simulink model "Synch_gen_model_full_order"  (R2013a)
settings: Solver=ode23tb  StartTime=0.0  StopTime=10  FixedStep=0.01  MaxStep=0.0005  RelTol=1e-5  AbsTol=1e-4
values from neighbouring files (symbols this model uses):
  D = 0    [Gen_Init_SynFull_Order.m]
  deltag0 = angle(Uq0bar)    [Gen_Init_SynFull_Order.m]
  H = 2.86    [Gen_Init_SynFull_Order.m]
  Ra = 0.01    [Gen_Init_SynFull_Order.m]
  RL = uqg0/iq0    [Gen_Init_SynFull_Order.m]
  sid0 = xd*id0+Ufd0    [Gen_Init_SynFull_Order.m]
  sif0 = sid0 + (xdd/(xd-xdd))*Ufd0    [Gen_Init_SynFull_Order.m]
  sig0 = siq0    [Gen_Init_SynFull_Order.m]
  SigmaInv = 1/0.05    (= 20)    [Gen_Init_SynFull_Order.m]
  sih0 = sid0    [Gen_Init_SynFull_Order.m]
  sik0 = siq0    [Gen_Init_SynFull_Order.m]
  siq0 = xq*iq0    [Gen_Init_SynFull_Order.m]
  Tdd = 0.4    [Gen_Init_SynFull_Order.m]
  Tddd = 0.0259    [Gen_Init_SynFull_Order.m]
  Tm = Te0    [Gen_Init_SynFull_Order.m]
  Tqd = 0.1073    [Gen_Init_SynFull_Order.m]
  Tqdd = 0.0463    [Gen_Init_SynFull_Order.m]
  Tswitch = input('Enter the time at which Genarator is synchronized: ')    [Gen_Init_SynFull_Order.m]
  Ufd0 = Uq0-(xd-xq)*id0    [Gen_Init_SynFull_Order.m]
  w0 = 50*2*pi    (= 314.159265359)    [Gen_Init_SynFull_Order.m]
  W0init = 1    [Gen_Init_SynFull_Order.m]
  wB = 50*2*pi    (= 314.159265359)    [Gen_Init_SynFull_Order.m]
  xd = 1.79    [Gen_Init_SynFull_Order.m]
  xdd = 0.169    [Gen_Init_SynFull_Order.m]
  xddd = 0.135    [Gen_Init_SynFull_Order.m]
  xfl = (xd*xdd)/(xd-xdd)    (= 0.186619370759)    [Gen_Init_SynFull_Order.m]
  xq = 1.71    [Gen_Init_SynFull_Order.m]
  xqd = 0.228    [Gen_Init_SynFull_Order.m]
  xqdd = 0.2    [Gen_Init_SynFull_Order.m]
  Ymat = inv(Zmat)    [Gen_Init_SynFull_Order.m]
settings Model: Creator=Korai  LastModifiedBy=Korai
settings RTWCC: TargetLang=C++

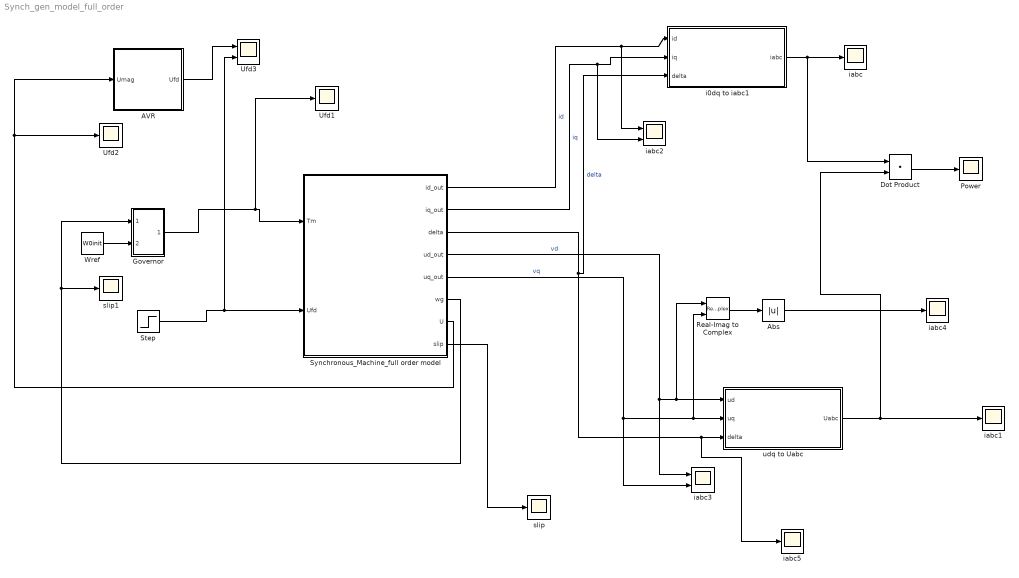
== system Synch_gen_model_full_order ==
  AVR : Subsystem
  Abs : Abs
  Dot Product : DotProduct  InputSameDT=on  OutDataTypeStr=Inherit: Inherit via internal rule
  Governor : Subsystem
  Power : Scope
      settings: YMin=0.0095  YMax=0.0105  SaveName=ScopeData5
  Real-Imag to Complex : RealImagToComplex
  Step : Step  Time=0  After=Ufd0  SampleTime=0
  Synchronous_Machine_full order model : Subsystem
  Ufd1 : Scope
      settings: YMin=-0.55  YMax=0.55  SaveName=ScopeData11
  Ufd2 : Scope
      settings: SaveName=ScopeData13
  Ufd3 : Scope  NumInputPorts=2
      settings: YMin=-3e-05~1.03987  YMax=2.25e-05~1.14933  SaveName=ScopeData16
  Wref : Constant  Value=W0init
  i0dq to iabc1 : Subsystem
  iabc{,1,4..5} (4 alike) : Scope
      iabc settings: YMin=-7  YMax=7
      iabc1 settings: YMin=-0.9  YMax=0.9  SaveName=ScopeData2
      iabc4 settings: YMin=0.95  YMax=1.05  SaveName=ScopeData23
      iabc5 settings: YMin=-0.9  YMax=0.9  SaveName=ScopeData25
  iabc2 : Scope  NumInputPorts=2
      settings: ShowLegends=on  YMin=-0.0004865~0.02665  YMax=-0.000475~0.0272  SaveName=ScopeData9
  iabc3 : Scope  NumInputPorts=2
      settings: ShowLegends=on  YMin=-0.0184~0.99983  YMax=-0.0166~0.999862  SaveName=ScopeData10
  slip : Scope
      settings: SaveName=ScopeData12
  slip1 : Scope
      settings: SaveName=ScopeData24
  udq to Uabc : Subsystem
  wires:
  i0dq to iabc1/1(iabc) -> iabc/1, Dot Product/1
  udq to Uabc/1(Uabc) -> Dot Product/2, iabc1/1
  Dot Product/1 -> Power/1
  Synchronous_Machine_full order model/3(delta) -> i0dq to iabc1/3(delta), iabc5/1, udq to Uabc/3(delta)  "delta"
  Synchronous_Machine_full order model/1(id_out) -> i0dq to iabc1/1(id), iabc2/1  "id"
  Synchronous_Machine_full order model/2(iq_out) -> i0dq to iabc1/2(iq), iabc2/2  "iq"
  Synchronous_Machine_full order model/4("ud_out ") -> Real-Imag to Complex/1, udq to Uabc/1(ud), iabc3/1  "vd"
  Synchronous_Machine_full order model/5(uq_out) -> Real-Imag to Complex/2, udq to Uabc/2(uq), iabc3/2  "vq"
  Synchronous_Machine_full order model/6(wg) -> slip1/1, Governor/1(wpu)
  Wref/1 -> Governor/2(w_ref)
  Synchronous_Machine_full order model/7(U) -> AVR/1(Umag), Ufd2/1
  Synchronous_Machine_full order model/8(slip) -> slip/1
  Governor/1(Tm) -> Ufd1/1, Synchronous_Machine_full order model/1(Tm)
  Real-Imag to Complex/1 -> Abs/1
  Abs/1 -> iabc4/1
  AVR/1(Ufd) -> Ufd3/1
  Step/1 -> Ufd3/2, Synchronous_Machine_full order model/2(Ufd)

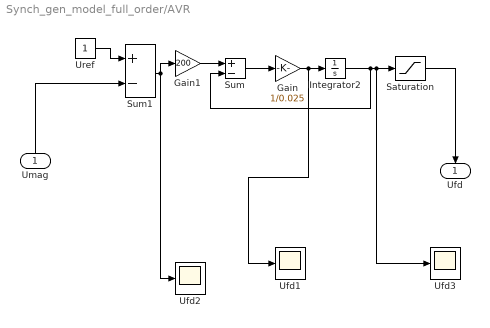
== system Synch_gen_model_full_order/AVR ==
  Umag : Inport
  Gain : Gain  Gain=1/0.025  SaturateOnIntegerOverflow=on  OutDataTypeStr=Inherit: Same as input  ParamDataTypeStr=Inherit: Same as input
  Gain1 : Gain  Gain=200  SaturateOnIntegerOverflow=on  OutDataTypeStr=Inherit: Same as input  ParamDataTypeStr=Inherit: Same as input
  Integrator2 : Integrator  InitialCondition=Ufd0
  Saturation : Saturate  UpperLimit=6  LowerLimit=-6
  Sum : Sum  Inputs=+-  SaturateOnIntegerOverflow=on  InputSameDT=on  OutDataTypeStr=Inherit: Same as first input
  Sum1 : Sum  Inputs=+-  SaturateOnIntegerOverflow=on  InputSameDT=on  OutDataTypeStr=Inherit: Same as first input
  Ufd1 : Scope
      settings: YMin=-550  YMax=550  SaveName=ScopeData19
  Ufd2 : Scope
      settings: YMin=-0.08  YMax=0.07  SaveName=ScopeData20
  Ufd3 : Scope
      settings: YMin=-2.75  YMax=1  SaveName=ScopeData18
  Uref : Constant
  Ufd : Outport
  wires:
  Gain/1 -> Ufd1/1, Integrator2/1
  Saturation/1 -> Ufd/1
  Sum/1 -> Gain/1
  Uref/1 -> Sum1/1
  Gain1/1 -> Sum/1
  Integrator2/1 -> Sum/2, Ufd3/1, Saturation/1
  Sum1/1 -> Gain1/1, Ufd2/1
  Umag/1 -> Sum1/2

== system Synch_gen_model_full_order/Governor ==
  wpu : Inport
  w_ref : Inport  Port=2
  Gain : Gain  Gain=1/0.01  SaturateOnIntegerOverflow=on  OutDataTypeStr=Inherit: Same as input  ParamDataTypeStr=Inherit: Same as input
  Gain15 : Gain  Gain=SigmaInv  SaturateOnIntegerOverflow=on  OutDataTypeStr=Inherit: Same as input  ParamDataTypeStr=Inherit: Same as input
  Integrator : Integrator  InitialCondition=Tm
  Sum : Sum  Inputs=+-  SaturateOnIntegerOverflow=on  InputSameDT=on  OutDataTypeStr=Inherit: Same as first input
  Sum1 : Sum  SaturateOnIntegerOverflow=on  InputSameDT=on  OutDataTypeStr=Inherit: Same as first input
  Sum8 : Sum  Inputs=+-  SaturateOnIntegerOverflow=on  InputSameDT=on  OutDataTypeStr=Inherit: Same as first input
  Tm0 : Constant  Value=Tm
  Tm : Outport
  wires:
  w_ref/1 -> Sum8/1
  Sum8/1 -> Gain15/1
  wpu/1 -> Sum8/2
  Sum/1 -> Gain/1
  Gain/1 -> Integrator/1
  Integrator/1 -> Sum/2, Tm/1
  Gain15/1 -> Sum1/2
  Sum1/1 -> Sum/1
  Tm0/1 -> Sum1/1

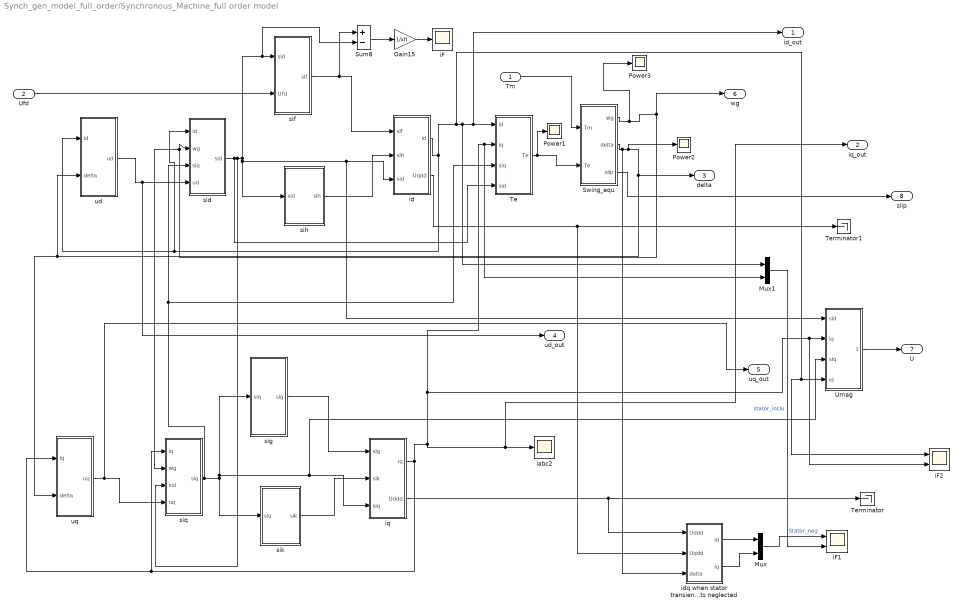
== system Synch_gen_model_full_order/Synchronous_Machine_full order model ==
  Tm : Inport
  Ufd : Inport  Port=2
  Gain15 : Gain  Gain=1/xfl  SaturateOnIntegerOverflow=on  OutDataTypeStr=Inherit: Same as input  ParamDataTypeStr=Inherit: Same as input
  Mux : Mux  Inputs=2
  Mux1 : Mux  Inputs=2
  Power1 : Scope
      settings: YMin=0.010195  YMax=0.01023  SaveName=ScopeData6
  Power2 : Scope
      settings: YMin=0.82  YMax=0.885  SaveName=ScopeData7
  Power3 : Scope
      settings: YMin=0.95  YMax=1.05  SaveName=ScopeData8
  Sum8 : Sum  Inputs=+-  SaturateOnIntegerOverflow=on  InputSameDT=on  OutDataTypeStr=Inherit: Same as first input
  "Swing_equ " : Subsystem
  Te : Subsystem
  Terminator : Terminator
  Terminator1 : Terminator
  Umag : Subsystem
  iF : Scope
      settings: SaveName=ScopeData4
  iF1 : Scope  NumInputPorts=2
      settings: ShowLegends=on  YMin=-17.5~-25  YMax=7.5~12.5  SaveName=ScopeData14
  iF2 : Scope  NumInputPorts=2
      settings: YMin=-0.191~0.190025  YMax=-0.189~0.1905  SaveName=ScopeData15
  iabc2 : Scope
      settings: YMin=0.0054  YMax=0.00645  SaveName=ScopeData3
  id : Subsystem
  idq when stator transients neglected : Subsystem
  iq : Subsystem
  sid : Subsystem
  sif : Subsystem
  sig : Subsystem
  sih : Subsystem
  sik : Subsystem
  siq : Subsystem
  ud : Subsystem
  uq : Subsystem
  id_out : Outport
  iq_out : Outport  Port=2
  delta : Outport  Port=3
  "ud_out " : Outport  Port=4
  uq_out : Outport  Port=5
  wg : Outport  Port=6
  U : Outport  Port=7
  slip : Outport  Port=8
  wires:
  iq/2(Uddd) -> idq when stator transients neglected/1(Uddd), Terminator/1
  id/1(id) -> Umag/4(id), iF2/1, Mux1/1, id_out/1, Te/1(id), sid/1(id), ud/1(id)
  sif/1(sif) -> Sum8/1, id/1(sif)
  sih/1(sih) -> id/2(sih)
  sid/1(sid) -> Te/4(sid), siq/3(sid), Sum8/2, sif/1(sid), sih/1(sid), Umag/1(sid), id/3(sid)
  iq/1(iq) -> uq/1(iq), siq/1(iq), Mux1/2, Te/2(iq), iF2/2, Umag/2(iq), iq_out/1, iabc2/1
  Gain15/1 -> iF/1
  Tm/1 -> "Swing_equ "/1(Tm)
  Sum8/1 -> Gain15/1
  id/2(Uqdd) -> Terminator1/1, idq when stator transients neglected/2(Uqdd)
  sik/1(sik) -> iq/2(sik)
  Te/1(Te) -> "Swing_equ "/2(Te), Power1/1
  "Swing_equ "/1(wg) -> Power3/1, siq/2(wg), sid/2(wg), wg/1
  "Swing_equ "/2(delta) -> idq when stator transients neglected/3(delta), Power2/1, delta/1, uq/2(delta), ud/2(delta)
  sig/1(sig) -> iq/1(sig)
  siq/1(siq) -> Te/3(siq), sid/3(siq), Umag/3(siq), iq/3(siq), sig/1(siq), sik/1(siq)
  Ufd/1 -> sif/2(Ufd)
  Umag/1(Umag) -> U/1
  "Swing_equ "/3(slip) -> slip/1
  ud/1(ud) -> "ud_out "/1, sid/4(ud)
  uq/1(uq) -> uq_out/1, siq/4(uq)
  idq when stator transients neglected/1(id) -> Mux/1
  idq when stator transients neglected/2(iq) -> Mux/2
  Mux/1 -> iF1/1  "Stator_neg"
  Mux1/1 -> iF1/2  "stator_inclu"

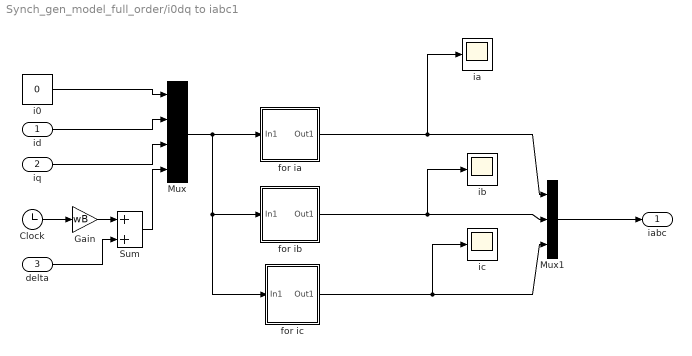
== system Synch_gen_model_full_order/i0dq to iabc1 ==
  id : Inport
  iq : Inport  Port=2
  delta : Inport  Port=3
  Clock : Clock
  Gain : Gain  Gain=wB  SaturateOnIntegerOverflow=on  OutDataTypeStr=Inherit: Same as input  ParamDataTypeStr=Inherit: Same as input
  Mux : Mux
  Mux1 : Mux  Inputs=3
  Sum : Sum  Inputs=|++  SaturateOnIntegerOverflow=on  InputSameDT=on  OutDataTypeStr=Inherit: Same as first input
  for ia : Subsystem
  for ib : Subsystem
  for ic : Subsystem
  i0 : Constant  Value=0
  ia : Scope
  ib : Scope
  ic : Scope
  iabc : Outport
  wires:
  i0/1 -> Mux/1
  Sum/1 -> Mux/4
  Clock/1 -> Gain/1
  Gain/1 -> Sum/1
  delta/1 -> Sum/2
  Mux/1 -> for ic/1(In1), for ib/1(In1), for ia/1(In1)
  Mux1/1 -> iabc/1
  iq/1 -> Mux/3
  id/1 -> Mux/2
  for ic/1(Out1) -> ic/1, Mux1/3
  for ib/1(Out1) -> ib/1, Mux1/2
  for ia/1(Out1) -> ia/1, Mux1/1

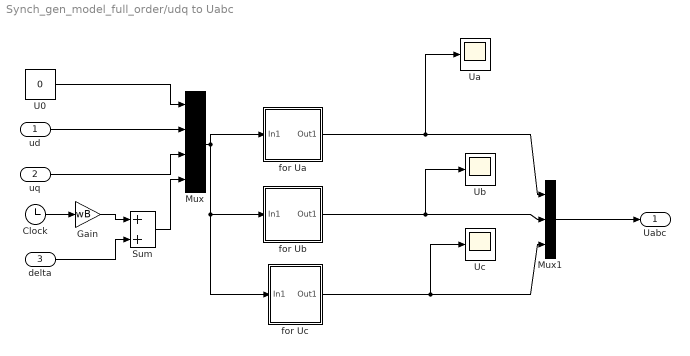
== system Synch_gen_model_full_order/udq to Uabc ==
  ud : Inport
  uq : Inport  Port=2
  delta : Inport  Port=3
  Clock : Clock
  Gain : Gain  Gain=wB  SaturateOnIntegerOverflow=on  OutDataTypeStr=Inherit: Same as input  ParamDataTypeStr=Inherit: Same as input
  Mux : Mux
  Mux1 : Mux  Inputs=3
  Sum : Sum  Inputs=|++  SaturateOnIntegerOverflow=on  InputSameDT=on  OutDataTypeStr=Inherit: Same as first input
  U0 : Constant  Value=0
  Ua : Scope
  Ub : Scope
  Uc : Scope
  for Ua : Subsystem
  for Ub : Subsystem
  for Uc : Subsystem
  Uabc : Outport
  wires:
  for Ua/1(Out1) -> Mux1/1, Ua/1
  for Ub/1(Out1) -> Mux1/2, Ub/1
  for Uc/1(Out1) -> Mux1/3, Uc/1
  U0/1 -> Mux/1
  ud/1 -> Mux/2
  uq/1 -> Mux/3
  Mux1/1 -> Uabc/1
  delta/1 -> Sum/2
  Clock/1 -> Gain/1
  Gain/1 -> Sum/1
  Sum/1 -> Mux/4
  Mux/1 -> for Ua/1(In1), for Ub/1(In1), for Uc/1(In1)

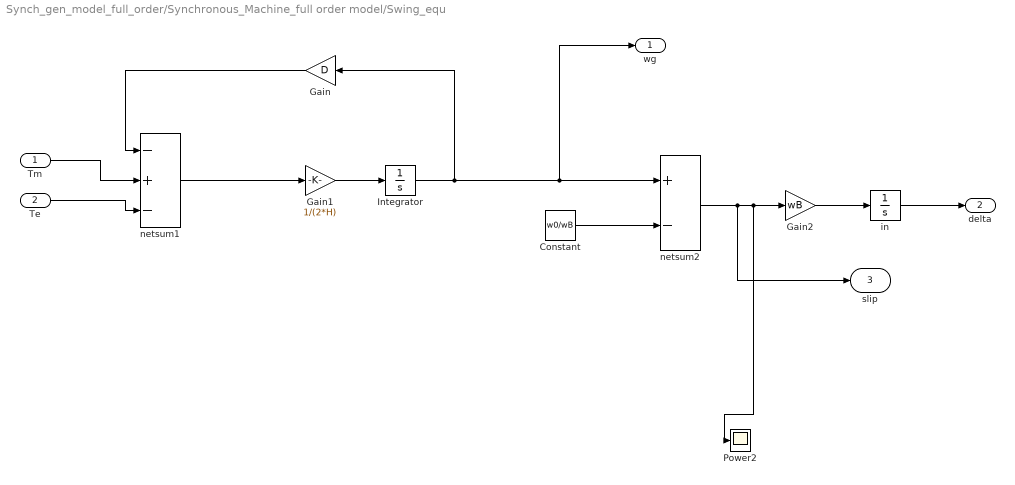
== system Synch_gen_model_full_order/Synchronous_Machine_full order model/Swing_equ  ==
  Tm : Inport
  Te : Inport  Port=2
  Constant : Constant  Value=w0/wB
  Gain : Gain  Gain=D
  Gain1 : Gain  Gain=1/(2*H)
  Gain2 : Gain  Gain=wB  SaturateOnIntegerOverflow=on  OutDataTypeStr=Inherit: Same as input  ParamDataTypeStr=Inherit: Same as input
  Integrator : Integrator  InitialCondition=W0init
  Power2 : Scope
      settings: YMin=0.82  YMax=0.885  SaveName=ScopeData26
  in : Integrator  InitialCondition=deltag0
  netsum1 : Sum  Inputs=-+-  SaturateOnIntegerOverflow=on  InputSameDT=on  OutDataTypeStr=Inherit: Same as first input
  netsum2 : Sum  Inputs=+-  SaturateOnIntegerOverflow=on  InputSameDT=on  OutDataTypeStr=Inherit: Same as first input
  wg : Outport
  delta : Outport  Port=2
  slip : Outport  Port=3
  wires:
  Te/1 -> netsum1/3
  Tm/1 -> netsum1/2
  Gain/1 -> netsum1/1
  netsum1/1 -> Gain1/1
  Gain1/1 -> Integrator/1
  Integrator/1 -> netsum2/1, wg/1, Gain/1
  Constant/1 -> netsum2/2
  Gain2/1 -> in/1
  in/1 -> delta/1
  netsum2/1 -> slip/1, Power2/1, Gain2/1

== system Synch_gen_model_full_order/Synchronous_Machine_full order model/Te ==
  id : Inport
  iq : Inport  Port=2
  siq : Inport  Port=3
  sid : Inport  Port=4
  Product : Product
  Product1 : Product
  netsum : Sum  Inputs=+-  SaturateOnIntegerOverflow=on  InputSameDT=on  OutDataTypeStr=Inherit: Same as first input
  Te : Outport
  wires:
  netsum/1 -> Te/1
  sid/1 -> Product/1
  iq/1 -> Product/2
  Product/1 -> netsum/1
  id/1 -> Product1/1
  siq/1 -> Product1/2
  Product1/1 -> netsum/2

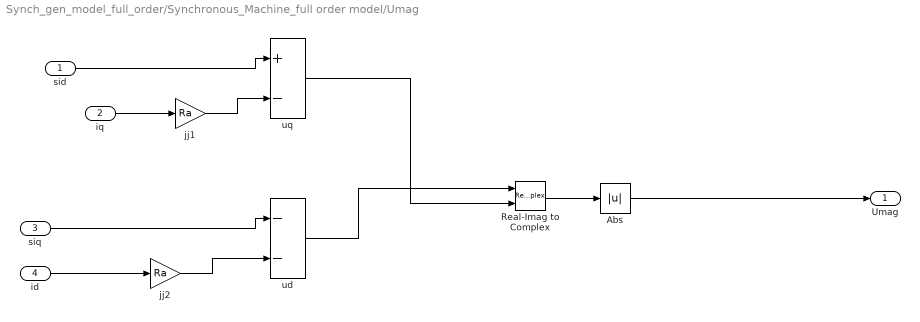
== system Synch_gen_model_full_order/Synchronous_Machine_full order model/Umag ==
  sid : Inport
  iq : Inport  Port=2
  siq : Inport  Port=3
  id : Inport  Port=4
  Abs : Abs
  Real-Imag to Complex : RealImagToComplex
  jj1 : Gain  Gain=Ra
  jj2 : Gain  Gain=Ra
  ud : Sum  Inputs=--  SaturateOnIntegerOverflow=on  InputSameDT=on  OutDataTypeStr=Inherit: Same as first input
  uq : Sum  Inputs=+-  SaturateOnIntegerOverflow=on  InputSameDT=on  OutDataTypeStr=Inherit: Same as first input
  Umag : Outport
  wires:
  sid/1 -> uq/1
  Abs/1 -> Umag/1
  iq/1 -> jj1/1
  jj1/1 -> uq/2
  siq/1 -> ud/1
  id/1 -> jj2/1
  jj2/1 -> ud/2
  uq/1 -> Real-Imag to Complex/2
  ud/1 -> Real-Imag to Complex/1
  Real-Imag to Complex/1 -> Abs/1

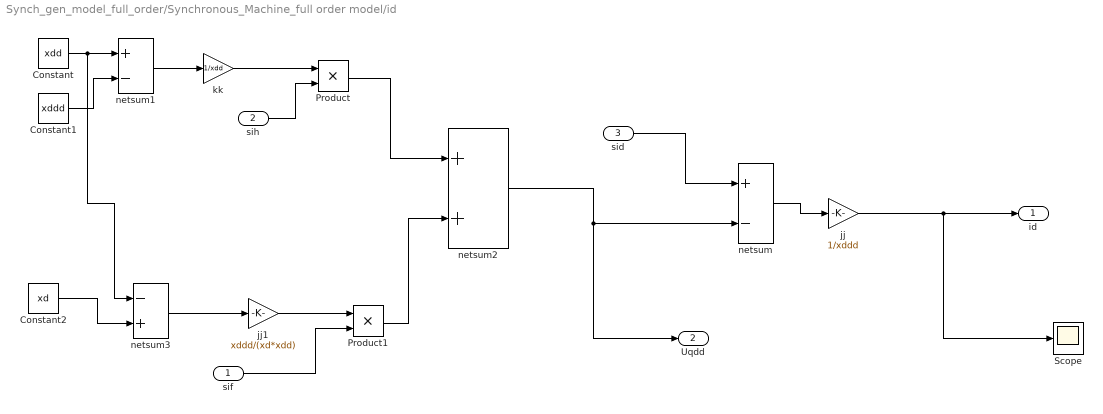
== system Synch_gen_model_full_order/Synchronous_Machine_full order model/id ==
  sif : Inport
  sih : Inport  Port=2
  sid : Inport  Port=3
  Constant : Constant  Value=xdd
  Constant1 : Constant  Value=xddd
  Constant2 : Constant  Value=xd
  Product : Product
  Product1 : Product
  Scope : Scope
      settings: SaveName=ScopeData29
  jj : Gain  Gain=1/xddd
  jj1 : Gain  Gain=xddd/(xd*xdd)
  kk : Gain  Gain=1/xdd
  netsum : Sum  Inputs=+-  SaturateOnIntegerOverflow=on  InputSameDT=on  OutDataTypeStr=Inherit: Same as first input
  netsum1 : Sum  Inputs=+-  SaturateOnIntegerOverflow=on  InputSameDT=on  OutDataTypeStr=Inherit: Same as first input
  netsum2 : Sum  SaturateOnIntegerOverflow=on  InputSameDT=on  OutDataTypeStr=Inherit: Same as first input
  netsum3 : Sum  Inputs=-+  SaturateOnIntegerOverflow=on  InputSameDT=on  OutDataTypeStr=Inherit: Same as first input
  id : Outport
  Uqdd : Outport  Port=2
  wires:
  Constant/1 -> netsum3/1, netsum1/1
  Constant1/1 -> netsum1/2
  netsum1/1 -> kk/1
  kk/1 -> Product/1
  sih/1 -> Product/2
  Product/1 -> netsum2/1
  Constant2/1 -> netsum3/2
  netsum3/1 -> jj1/1
  jj1/1 -> Product1/1
  sif/1 -> Product1/2
  Product1/1 -> netsum2/2
  netsum2/1 -> netsum/2, Uqdd/1
  sid/1 -> netsum/1
  netsum/1 -> jj/1
  jj/1 -> Scope/1, id/1

== system Synch_gen_model_full_order/Synchronous_Machine_full order model/idq when stator transients neglected ==
  Uddd : Inport
  Uqdd : Inport  Port=2
  delta : Inport  Port=3
  Demux : Demux  Outputs=2
  Mux1 : Mux  Inputs=2
  Synchronize : Subsystem
  id1 : Scope
      settings: YMin=0.165532  YMax=0.165582
  iq1 : Scope
      settings: YMin=0.165532  YMax=0.165582
  id : Outport
  iq : Outport  Port=2
  wires:
  delta/1 -> Synchronize/2(delta)
  Uddd/1 -> Mux1/1
  Uqdd/1 -> Mux1/2
  Mux1/1 -> Synchronize/1(UdddUqdd)
  Demux/1 -> id/1, id1/1
  Demux/2 -> iq/1, iq1/1
  Synchronize/1(idq) -> Demux/1

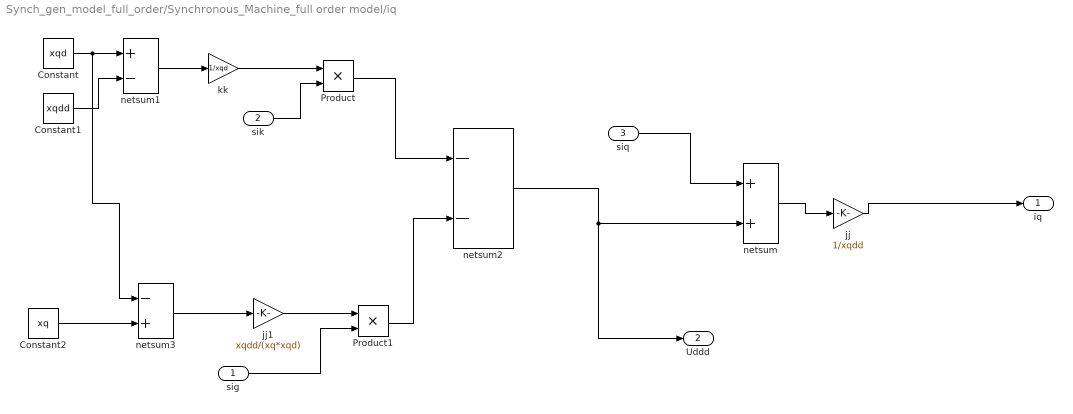
== system Synch_gen_model_full_order/Synchronous_Machine_full order model/iq ==
  sig : Inport
  sik : Inport  Port=2
  siq : Inport  Port=3
  Constant : Constant  Value=xqd
  Constant1 : Constant  Value=xqdd
  Constant2 : Constant  Value=xq
  Product : Product
  Product1 : Product
  jj : Gain  Gain=1/xqdd
  jj1 : Gain  Gain=xqdd/(xq*xqd)
  kk : Gain  Gain=1/xqd
  netsum : Sum  SaturateOnIntegerOverflow=on  InputSameDT=on  OutDataTypeStr=Inherit: Same as first input
  netsum1 : Sum  Inputs=+-  SaturateOnIntegerOverflow=on  InputSameDT=on  OutDataTypeStr=Inherit: Same as first input
  netsum2 : Sum  Inputs=--  SaturateOnIntegerOverflow=on  InputSameDT=on  OutDataTypeStr=Inherit: Same as first input
  netsum3 : Sum  Inputs=-+  SaturateOnIntegerOverflow=on  InputSameDT=on  OutDataTypeStr=Inherit: Same as first input
  iq : Outport
  Uddd : Outport  Port=2
  wires:
  Constant/1 -> netsum3/1, netsum1/1
  Constant1/1 -> netsum1/2
  netsum1/1 -> kk/1
  kk/1 -> Product/1
  sik/1 -> Product/2
  Product/1 -> netsum2/1
  Constant2/1 -> netsum3/2
  netsum3/1 -> jj1/1
  jj1/1 -> Product1/1
  sig/1 -> Product1/2
  Product1/1 -> netsum2/2
  netsum2/1 -> netsum/2, Uddd/1
  siq/1 -> netsum/1
  netsum/1 -> jj/1
  jj/1 -> iq/1

== system Synch_gen_model_full_order/Synchronous_Machine_full order model/sid ==
  id : Inport
  wg : Inport  Port=2
  siq : Inport  Port=3
  ud : Inport  Port=4
  Integrator : Integrator  InitialCondition=sid0
  Product : Product
  Ra : Gain  Gain=Ra
  netsum : Sum  Inputs=---  SaturateOnIntegerOverflow=on  InputSameDT=on  OutDataTypeStr=Inherit: Same as first input
  wb : Gain  Gain=wB
  sid : Outport
  wires:
  Ra/1 -> netsum/3
  netsum/1 -> wb/1
  Integrator/1 -> sid/1
  wb/1 -> Integrator/1
  Product/1 -> netsum/2
  id/1 -> Ra/1
  wg/1 -> Product/2
  siq/1 -> Product/1
  ud/1 -> netsum/1

== system Synch_gen_model_full_order/Synchronous_Machine_full order model/sif ==
  sid : Inport
  Ufd : Inport  Port=2
  1 : Gain  Gain=xdd/(xd-xdd)
  Integrator : Integrator  InitialCondition=sif0
  iF : Scope
      settings: YMin=0.95  YMax=1.1  SaveName=ScopeData21
  iF1 : Scope
      settings: YMin=0.9575  YMax=0.9675  SaveName=ScopeData22
  netsum : Sum  SaturateOnIntegerOverflow=on  InputSameDT=on  OutDataTypeStr=Inherit: Same as first input
  netsum1 : Sum  Inputs=+-  SaturateOnIntegerOverflow=on  InputSameDT=on  OutDataTypeStr=Inherit: Same as first input
  tdd : Gain  Gain=1/Tdd
  sif : Outport
  wires:
  Integrator/1 -> netsum1/2, iF/1, sif/1
  tdd/1 -> Integrator/1
  sid/1 -> iF1/1, netsum/2
  Ufd/1 -> 1/1
  1/1 -> netsum/1
  netsum/1 -> netsum1/1
  netsum1/1 -> tdd/1

== system Synch_gen_model_full_order/Synchronous_Machine_full order model/sig ==
  siq : Inport
  Integrator : Integrator  InitialCondition=sig0
  netsum1 : Sum  Inputs=+-  SaturateOnIntegerOverflow=on  InputSameDT=on  OutDataTypeStr=Inherit: Same as first input
  tdd : Gain  Gain=1/Tqd
  sig : Outport
  wires:
  Integrator/1 -> netsum1/2, sig/1
  tdd/1 -> Integrator/1
  netsum1/1 -> tdd/1
  siq/1 -> netsum1/1

== system Synch_gen_model_full_order/Synchronous_Machine_full order model/sih ==
  sid : Inport
  Integrator : Integrator  InitialCondition=sih0
  netsum1 : Sum  Inputs=+-  SaturateOnIntegerOverflow=on  InputSameDT=on  OutDataTypeStr=Inherit: Same as first input
  tdd : Gain  Gain=1/Tddd
  sih : Outport
  wires:
  Integrator/1 -> netsum1/2, sih/1
  tdd/1 -> Integrator/1
  sid/1 -> netsum1/1
  netsum1/1 -> tdd/1

== system Synch_gen_model_full_order/Synchronous_Machine_full order model/sik ==
  siq : Inport
  Integrator : Integrator  InitialCondition=sik0
  netsum1 : Sum  Inputs=+-  SaturateOnIntegerOverflow=on  InputSameDT=on  OutDataTypeStr=Inherit: Same as first input
  tdd : Gain  Gain=1/Tqdd
  sik : Outport
  wires:
  Integrator/1 -> netsum1/2, sik/1
  tdd/1 -> Integrator/1
  siq/1 -> netsum1/1
  netsum1/1 -> tdd/1

== system Synch_gen_model_full_order/Synchronous_Machine_full order model/siq ==
  iq : Inport
  wg : Inport  Port=2
  sid : Inport  Port=3
  uq : Inport  Port=4
  Integrator : Integrator  InitialCondition=siq0
  Product : Product
  Ra : Gain  Gain=Ra
  netsum : Sum  Inputs=-+-  SaturateOnIntegerOverflow=on  InputSameDT=on  OutDataTypeStr=Inherit: Same as first input
  wb : Gain  Gain=wB
  siq : Outport
  wires:
  Ra/1 -> netsum/3
  netsum/1 -> wb/1
  Integrator/1 -> siq/1
  wb/1 -> Integrator/1
  Product/1 -> netsum/2
  iq/1 -> Ra/1
  wg/1 -> Product/2
  sid/1 -> Product/1
  uq/1 -> netsum/1

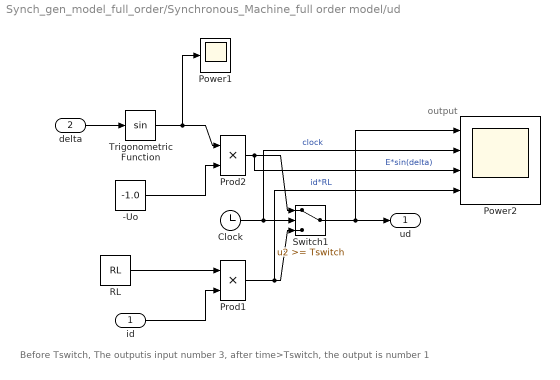
== system Synch_gen_model_full_order/Synchronous_Machine_full order model/ud ==
  note: Before Tswitch, The outputis input number 3, after time>Tswitch, the output is number 1
  note: output
  id : Inport
  delta : Inport  Port=2
  -Uo : Constant  Value=-1.0
  Clock : Clock
  Power1 : Scope
      settings: ShowLegends=on  YMin=-1  YMax=0.75  SaveName=ScopeData27
  Power2 : Scope  NumInputPorts=4
      settings: ShowLegends=on  YMin=-1~35~-1~-1750  YMax=0.75~85~1~250  SaveName=ScopeData17
  Prod1 : Product  SaturateOnIntegerOverflow=on  RndMeth=Zero  InputSameDT=on  OutDataTypeStr=Inherit: Same as first input
  Prod2 : Product  SaturateOnIntegerOverflow=on  RndMeth=Zero  InputSameDT=on  OutDataTypeStr=Inherit: Same as first input
  RL : Constant  Value=RL
  Switch1 : Switch  Threshold=Tswitch  SaturateOnIntegerOverflow=on  InputSameDT=on
  Trigonometric Function : Trigonometry
  ud : Outport
  wires:
  id/1 -> Prod1/2
  RL/1 -> Prod1/1
  Prod1/1 -> Power2/4, Switch1/3  "id*RL"
  Clock/1 -> Power2/2, Switch1/2  "clock"
  Switch1/1 -> Power2/1, ud/1
  Prod2/1 -> Switch1/1, Power2/3  "E*sin(delta)"
  Trigonometric Function/1 -> Prod2/1, Power1/1
  delta/1 -> Trigonometric Function/1
  -Uo/1 -> Prod2/2

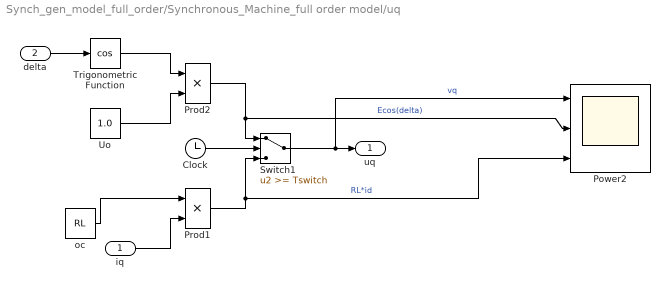
== system Synch_gen_model_full_order/Synchronous_Machine_full order model/uq ==
  iq : Inport
  delta : Inport  Port=2
  Clock : Clock
  Power2 : Scope  NumInputPorts=3
      settings: ShowLegends=on  YMin=-1~35~-1  YMax=0.75~85~1  SaveName=ScopeData28
  Prod1 : Product  SaturateOnIntegerOverflow=on  RndMeth=Zero  InputSameDT=on  OutDataTypeStr=Inherit: Same as first input
  Prod2 : Product  SaturateOnIntegerOverflow=on  RndMeth=Zero  InputSameDT=on  OutDataTypeStr=Inherit: Same as first input
  Switch1 : Switch  Threshold=Tswitch  SaturateOnIntegerOverflow=on  InputSameDT=on
  Trigonometric Function : Trigonometry  Operator=cos
  Uo : Constant  Value=1.0
  oc : Constant  Value=RL
  uq : Outport
  wires:
  Uo/1 -> Prod2/2
  delta/1 -> Trigonometric Function/1
  Trigonometric Function/1 -> Prod2/1
  Prod2/1 -> Power2/2, Switch1/1  "Ecos(delta)"
  Switch1/1 -> Power2/1, uq/1  "vq"
  Clock/1 -> Switch1/2
  Prod1/1 -> Switch1/3, Power2/3  "RL*id"
  oc/1 -> Prod1/1
  iq/1 -> Prod1/2

== system Synch_gen_model_full_order/i0dq to iabc1/for ia ==
  In1 : Inport
  Exp_Va : Fcn  Expr=sqrt(1/2)*(u[1])+u[2]*cos(u[4])+u[3]*sin(u[4])
  G : Gain  Gain=sqrt(2/3)  SaturateOnIntegerOverflow=on  OutDataTypeStr=Inherit: Same as input  ParamDataTypeStr=Inherit: Same as input
  Out1 : Outport
  wires:
  G/1 -> Out1/1
  In1/1 -> Exp_Va/1
  Exp_Va/1 -> G/1

== system Synch_gen_model_full_order/i0dq to iabc1/for ib ==
  In1 : Inport
  Exp_Vb : Fcn  Expr=sqrt(1/2)*(u[1])+u[2]*cos(u[4]-2*pi/3)+u[3]*sin(u[4]-2*pi/3)
  G1 : Gain  Gain=sqrt(2/3)  SaturateOnIntegerOverflow=on  OutDataTypeStr=Inherit: Same as input  ParamDataTypeStr=Inherit: Same as input
  Out1 : Outport
  wires:
  G1/1 -> Out1/1
  In1/1 -> Exp_Vb/1
  Exp_Vb/1 -> G1/1

== system Synch_gen_model_full_order/i0dq to iabc1/for ic ==
  In1 : Inport
  Exp_Vc : Fcn  Expr=sqrt(1/2)*(u[1])+u[2]*cos(u[4]+2*pi/3)+u[3]*sin(u[4]+2*pi/3)
  G2 : Gain  Gain=sqrt(2/3)  SaturateOnIntegerOverflow=on  OutDataTypeStr=Inherit: Same as input  ParamDataTypeStr=Inherit: Same as input
  Out1 : Outport
  wires:
  G2/1 -> Out1/1
  In1/1 -> Exp_Vc/1
  Exp_Vc/1 -> G2/1

== system Synch_gen_model_full_order/udq to Uabc/for Ua ==
  In1 : Inport
  Exp_Va : Fcn  Expr=sqrt(1/2)*(u[1])+u[2]*cos(u[4])+u[3]*sin(u[4])
  G : Gain  Gain=sqrt(2/3)  SaturateOnIntegerOverflow=on  OutDataTypeStr=Inherit: Same as input  ParamDataTypeStr=Inherit: Same as input
  Out1 : Outport
  wires:
  Exp_Va/1 -> G/1
  In1/1 -> Exp_Va/1
  G/1 -> Out1/1

== system Synch_gen_model_full_order/udq to Uabc/for Ub ==
  In1 : Inport
  Exp_Vb : Fcn  Expr=sqrt(1/2)*(u[1])+u[2]*cos(u[4]-2*pi/3)+u[3]*sin(u[4]-2*pi/3)
  G1 : Gain  Gain=sqrt(2/3)  SaturateOnIntegerOverflow=on  OutDataTypeStr=Inherit: Same as input  ParamDataTypeStr=Inherit: Same as input
  Out1 : Outport
  wires:
  Exp_Vb/1 -> G1/1
  In1/1 -> Exp_Vb/1
  G1/1 -> Out1/1

== system Synch_gen_model_full_order/udq to Uabc/for Uc ==
  In1 : Inport
  Exp_Vc : Fcn  Expr=sqrt(1/2)*(u[1])+u[2]*cos(u[4]+2*pi/3)+u[3]*sin(u[4]+2*pi/3)
  G2 : Gain  Gain=sqrt(2/3)  SaturateOnIntegerOverflow=on  OutDataTypeStr=Inherit: Same as input  ParamDataTypeStr=Inherit: Same as input
  Out1 : Outport
  wires:
  Exp_Vc/1 -> G2/1
  In1/1 -> Exp_Vc/1
  G2/1 -> Out1/1

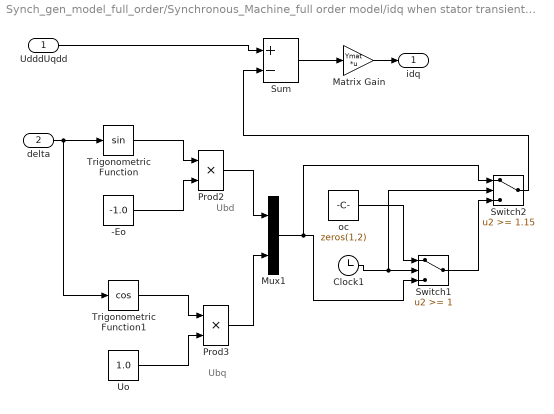
== system Synch_gen_model_full_order/Synchronous_Machine_full order model/idq when stator transients neglected/Synchronize ==
  note: Ubd
  note: Ubq
  UdddUqdd : Inport
  delta : Inport  Port=2
  -Eo : Constant  Value=-1.0
  Clock1 : Clock
  Matrix Gain : Gain  Gain=Ymat  Multiplication=Matrix(K*u)  SaturateOnIntegerOverflow=on  OutDataTypeStr=Inherit: Same as input  ParamDataTypeStr=Inherit: Same as input
  Mux1 : Mux  Inputs=2
  Prod2 : Product  SaturateOnIntegerOverflow=on  RndMeth=Zero  InputSameDT=on  OutDataTypeStr=Inherit: Same as first input
  Prod3 : Product  SaturateOnIntegerOverflow=on  RndMeth=Zero  InputSameDT=on  OutDataTypeStr=Inherit: Same as first input
  Sum : Sum  Inputs=+-  SaturateOnIntegerOverflow=on  InputSameDT=on  OutDataTypeStr=Inherit: Same as first input
  Switch1 : Switch  Threshold=1  SaturateOnIntegerOverflow=on  InputSameDT=on
  Switch2 : Switch  Threshold=1.15  SaturateOnIntegerOverflow=on  InputSameDT=on
  Trigonometric Function : Trigonometry
  Trigonometric Function1 : Trigonometry  Operator=cos
  Uo : Constant  Value=1.0
  oc : Constant  Value=zeros(1,2)
  idq : Outport
  wires:
  Trigonometric Function/1 -> Prod2/1
  -Eo/1 -> Prod2/2
  Uo/1 -> Prod3/2
  Trigonometric Function1/1 -> Prod3/1
  delta/1 -> Trigonometric Function/1, Trigonometric Function1/1
  Prod2/1 -> Mux1/1
  Prod3/1 -> Mux1/2
  UdddUqdd/1 -> Sum/1
  Sum/1 -> Matrix Gain/1
  Matrix Gain/1 -> idq/1
  oc/1 -> Switch1/1
  Clock1/1 -> Switch1/2, Switch2/2
  Switch1/1 -> Switch2/3
  Mux1/1 -> Switch1/3, Switch2/1
  Switch2/1 -> Sum/2
